simulink model "px4demo_ADC_example"  (R2017b)
settings: Solver=FixedStepAuto  StartTime=0.0  StopTime=inf  RelTol=1e-3  EnableMultiTasking=on
libraries: pixhawk_slib_ADC_serial x1
Description:
  | PX4 PSP Demo: ADC Block
  | 
  | Select the different ADC channels through the options in the block. This block was written as a system object. System objects are another alternate method of block authoring. The source code is written as MATLAB class.
  | 
  | To view the source code, a link is provided in the block description.
  | 
  | NOTE: This model is to be demosntrated in external mode. An alternative to being able to view these values without external mode is
  | to modify this example to print the signals to the Nuttshell terminal using the print block
settings Model: SimulationMode=external  Creator=darenlee  LastModifiedBy=skuznick
settings SolverCC: PositivePriorityOrder=on
settings DataIOCC: LimitDataPoints=on
settings OptimizationCC: DefaultParameterBehavior=Inlined  LifeSpan=1  MaxStackSize=64
settings DebuggingCC: AllowSymbolicDim=off  SFUnexpectedBacktrackingDiag=warning  SFNoUnconditionalDefaultTransitionDiag=warning  SFExecutionAtInitializationDiag=none
settings HardwareCC: ProdBitPerPointer=32  ProdBitPerSizeT=32  ProdBitPerPtrDiffT=32  ProdLargestAtomicInteger=Long  ProdLargestAtomicFloat=Double  ProdWordSize=32  ProdHWDeviceType=ARM Compatible->ARM Cortex
settings ModelReferenceCC: PropagateSignalLabelsOutOfModel=off
settings SFSimCC: MATLABDynamicMemAlloc=off
settings RTWCC: SystemTargetFile=ert.tlc  HardwareBoard=Pixhawk PX4  TemplateMakefile=ert_default_tmf  GenerateReport=on  Toolchain=Pixhawk Toolchain  IncludeHyperlinkInReport=on  LaunchReport=on  GenerateTraceInfo=on  GenerateTraceReport=on  GenerateTraceReportSl=on  GenerateTraceReportSf=on  GenerateTraceReportEml=on
settings CodeAppCC: ForceParamTrailComments=on  IgnoreCustomStorageClasses=off  OperatorAnnotations=on  StateflowObjectComments=on  MATLABSourceComments=on
settings ERTTargetCC: MultiwordLength=2048  ExtMode=on  ExtModeTransport=1  ExtModeMexFile=ext_serial_win32_comm  ExtModeMexArgs=1 7 115200  InlinedParameterPlacement=NonHierarchical  ERTCustomFileTemplate=px4_codertarget_file_process.tlc  ConvertIfToSwitch=off  SuppressUnreachableDefaultCases=off
settings ConfigComp: CovMetricSettings=dw  CovHtmlReporting=on  CovSaveCumulativeToWorkspaceVar=on  CovSaveSingleToWorkspaceVar=on  CovExternalEMLEnable=off

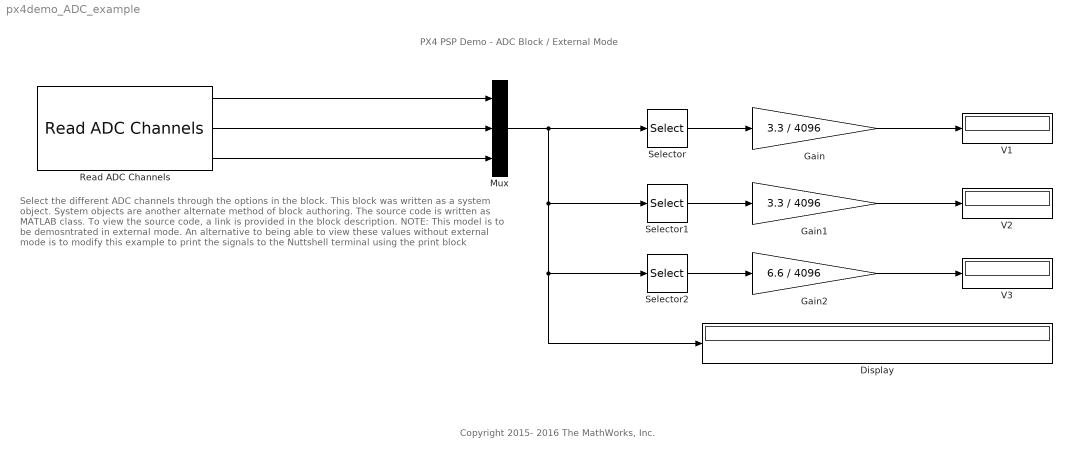
== system px4demo_ADC_example ==
  note: Select the different ADC channels through the options in the block. This block was written as a system object. System objects are another alternate method of block authoring. The source code is written as MATLAB class.
      |
      | To view the source code, a link is provided in the block description.
      |
      | NOTE: This model is to be demosntrated in external mode. An alternative to being able to view these values without external mode is
      | to modify this example to print the signals to the Nuttshell terminal using the print block
  note: PX4 PSP Demo - ADC Block / External Mode
  note: Copyright 2015- 2016 The MathWorks, Inc.
  Display : Display
  Gain : Gain  Gain=3.3 / 4096  ParamDataTypeStr=single  OutDataTypeStr=single
  Gain1 : Gain  Gain=3.3 / 4096  ParamDataTypeStr=single  OutDataTypeStr=single
  Gain2 : Gain  Gain=6.6 / 4096  ParamDataTypeStr=single  OutDataTypeStr=single
  Mux : Mux  Inputs=3
  Read ADC Channels : pixhawk_slib_ADC_serial/Read ADC Channels  ADC_Channel_3_3_1=on  ADC_Channel_3_3_2=on  ADC_Channel_6_6=on  SampleTime=0.1  SimulateUsing=Code generation
      settings: SourceProductName=Pixhawk Target Blocks
  Selector : Selector  InputPortWidth=3  IndexOptions=Index vector (dialog)  Indices=[1]  OutputSizes=1
  Selector1 : Selector  InputPortWidth=3  IndexOptions=Index vector (dialog)  Indices=[2]  OutputSizes=1
  Selector2 : Selector  InputPortWidth=3  IndexOptions=Index vector (dialog)  Indices=[3]  OutputSizes=1
  V1 : Display
  V2 : Display
  V3 : Display
  wires:
  Selector/1 -> Gain/1
  Gain/1 -> V1/1
  Selector1/1 -> Gain1/1
  Gain1/1 -> V2/1
  Selector2/1 -> Gain2/1
  Gain2/1 -> V3/1
  Read ADC Channels/1 -> Mux/1
  Mux/1 -> Display/1, Selector2/1, Selector1/1, Selector/1
  Read ADC Channels/2 -> Mux/2
  Read ADC Channels/3 -> Mux/3
